simulink model "MODULACIONFM"  (R2019a)
settings: Solver=VariableStepAuto  StartTime=0.0  StopTime=0.5  RelTol=1e-3
settings Model: Creator=JORGE  LastModifiedBy=JORGE

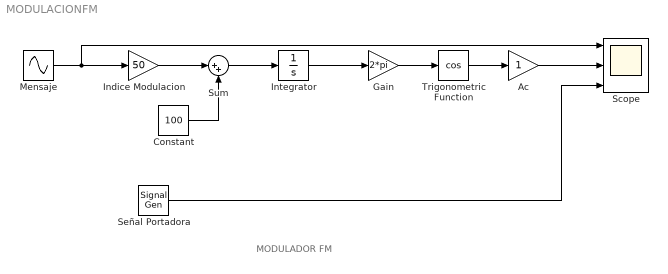
== system MODULACIONFM ==
  note: MODULADOR FM
  Ac : Gain
  "Constant " : Constant  Value=100
  "Gain " : Gain  Gain=2*pi
  "Indice Modulacion " : Gain  Gain=50
  "Integrator " : Integrator
  Mensaje : Sin  Frequency=2*pi*10  SampleTime=1/1000
  Scope : Scope  NumInputPorts=3
  Señal Portadora : SignalGenerator  Frequency=2*pi*50  Units=rad/sec
  Sum : Sum  Inputs=|++
  "Trigonometric Function " : Trigonometry  Operator=cos
  wires:
  Mensaje/1 -> Scope/1, "Indice Modulacion "/1
  "Indice Modulacion "/1 -> Sum/1
  Sum/1 -> "Integrator "/1
  "Integrator "/1 -> "Gain "/1
  "Gain "/1 -> "Trigonometric Function "/1
  "Trigonometric Function "/1 -> Ac/1
  Ac/1 -> Scope/2
  "Constant "/1 -> Sum/2
  Señal Portadora/1 -> Scope/3
